simulink model "full_sim123deleteme"  (R2020b)
settings: Solver=ode1be  StartTime=0.0  StopTime=inf  RelTol=1e-3
InitFcn:
  | % Clear persistent variables in callback
  | clear all;
  | 
  | track = gen_track;
  | map = double(rgb2gray(imread('map.png')));%'iSpaceMapV2.0_50dpi.png')))*100/255;
  | 
  | % Load config data automatically
  | load("config.mat");
StartFcn:
  | % The event listener triggers when the signal updates, so we can just monitor one of the signals.
  | blk1 = 'full_sim/GUI_update';
  | 
  | event = 'PostOutputs';
  | listener = @updateApp;
  | 
  | % Create the listener
  | h1 = add_exec_event_listener(blk1, event, listener);
model workspace (MAT data in the model file):
  ResetMode : string (value not decoded)
  initX = -0.39
  initY = 0.33
  initYaw = 3.14159265359
libraries: simulink_extras x10, simulink x8, dspnetwork x6, pid_lib x2, sldrtlib x1
(part 2 of 2)

== matlab function full_sim123deleteme/EV3/Sensor Input Block/MATLAB Function ==
  data: pos input; rcx output; rcy output; lcx output; lcy output
function [rcx,rcy,lcx,lcy] = fcn(pos)
x = pos(1) + 0.06*cos(pos(3));
y = pos(2) + 0.06*sin(pos(3));
xScale = 1979.37;
yScale = -1925.58;
% xScale = 349.2718;
% yScale = -339.591;
topYReal = 2.936;
leftXReal = -1.9;
topYPixel = 943;
leftXPixel = 972;
% topYPixel = 168;
% leftXPixel = 166;
%pixel coords
x = round(leftXPixel + (xScale * (x-leftXReal)));
y = round(topYPixel + (yScale * (y-topYReal)));
lcy = floor(y-34*cos(pos(3)));
lcx = floor(x-34*sin(pos(3)));
rcy = floor(y+34*cos(pos(3)));
rcx = floor(x+34*sin(pos(3)));
% lcy = floor(y-6*cos(pos(3)));
% lcx = floor(x-6*sin(pos(3)));
% rcy = floor(y+6*cos(pos(3)));
% rcx = floor(x+6*sin(pos(3)));

end

== matlab function full_sim123deleteme/EV3/Sensor Input Block/left circle check ==
  data: map input; rli output; x input; y input; r input
function rli = circle(map,x,y,r)
%x and y are the coordinates of the center of the circle
%r is the radius of the circle
region = map(y-r:y+r, x-r:x+r); %matlab indexes the opposite of images, select s square around the circle 
[MX,MY] = meshgrid(-r:r, -r:r);
mask = MX.^2 + MY.^2 <= r^2;
rli = sum(sum(region.*double(mask))) / sum(sum(mask));%sum(sum(mask));
rli = round(rli * .7 + 10);
end

== matlab function full_sim123deleteme/EV3/Sensor Input Block/right circle check ==
  data: map input; rli output; x input; y input; r input
function rli = circle(map,x,y,r)
%x and y are the coordinates of the center of the circle
%r is the radius of the circle
region = map(y-r:y+r, x-r:x+r); %matlab indexes the opposite of images, select s square around the circle 
[MX,MY] = meshgrid(-r:r, -r:r);
mask = MX.^2 + MY.^2 <= r^2;
rli = sum(sum(region.*double(mask))) / sum(sum(mask));%sum(sum(mask));
rli = round(rli*.7 + 10);
end

== matlab function full_sim123deleteme/EV3/Sensor Input Block/Ultra_Sonic_Fcn ==
  data: pos input; other_pos input; ultrasonic output; omega input
function ultrasonic = Ultra_Sonic_Fcn(pos,other_pos,omega)
%NOTE: Assumed that position is being sent is in meters 

range_bound = 10;   %to solve for the upper and lower bounds
range_bound1 = 10;
range_bound2 = 10;
range_bound3 = 10;
range_bound4 = 10;

upp = 60;
mid = 30;
low = 20; 

value1 = 10;
value2 = 20;
value3 = 30; 

%find the distance between the two EVs
dist = other_pos(1:2) - pos(1:2);
   

%solve for hypotenuse between two vehicles. 
    dist_sq = (dist(1))^2 + (dist(2))^2; 
    hyp = sqrt(dist_sq); 
    
%hyp is in m need to convert to cm
    hyp = hyp*100; 
    
%since the positions are at the midpoint of the vehicles and not at the edges
    hyp = hyp -14; 

 %increase bounds with relation to how far away vehicle is 
  if hyp<=upp && hyp>=mid
      range_bound1 = range_bound+value1; 
  elseif hyp<=mid && hyp>=low
      range_bound1 = range_bound+value2; 
  elseif hyp<low
      range_bound1 = range_bound+value3; 
  end 
     

%find the trajected angle for the head motor
angle = atan2(dist(2), dist(1)); 

%need to find the angle of the head motor in relation to the rotation of the actual EV
head_ang = angle - pos(3); 
head_ang = -rad2deg(head_ang); 

%keeps angle within +/- 180 degrees
head_angle = mod(head_ang+180, 360) - 180; 

%find bounding region range using angle and radius --> 255 cm 
%check to see if the position of the other vehicle is within that bounding
%range. It if it is send that distance, if not send in 255 cm 

lower_bound = rad2deg(angdiff(deg2rad(range_bound1),deg2rad(head_angle)));  %must wrap bounds so that they stay within +/- 180 degrees
upper_bound = rad2deg(angdiff(deg2rad(-range_bound1),deg2rad(head_angle))); 
omeg = mod(omega+180, 360)-180; 

% 
%  %((pos(1)<=-0.40)&& (pos(2)<= 1.7)&&(pos(2)>=1.5)) %parking spot 3
%     %finding midpoints
%     % spot 3:
%     % -.8906, 1.72
%     % -.4953, 1.62
%     % -.8977, 1.5883
%     % -.5013, 1.4928
%     
%    up1 = [-0.8906 ; 1.72]; 
%    lo1 = [-0.8977 ; 1.5883];
%     
%     mid_z1 = (1.72+ 1.5883)/2; 
%     mid_x1 = ((-0.8977)+(-0.8906))/2;
%     
%     
%     %find true midpoint
%     midpoint1 = [mid_x1; mid_z1];
%     %find distance and hypotenuese
%     d1 = midpoint1 - pos(1:2); 
%     d_sq1 = (d1(1))^2 + (d1(2))^2; 
%     hype1 = sqrt(d_sq1); 
%     
%     %send in ultrasonic and convert from m to cm 
%     u1 = hype1*100; 
%     
%      %increase bounds with relation to how far away vehicle is 
%   if u1<=upp && u1>=mid
%       range_bound2 = range_bound+value1; 
%   elseif u1<=mid && u1>=low
%       range_bound2 = range_bound+value2; 
%   elseif u1<low
%       range_bound2 = range_bound+value3; 
%   end 
%     
%         %Parking Spot 3
%   %find the distance between the two EVs
%    %dist1 = midpoint1 - pos(1:2);
%    up_dist1 = up1 - pos(1:2);
%    lo_dist1 = lo1 - pos(1:2); 
% 
% %find the trajected angle for the head motor
%  %angle1 = atan2(dist1(2), dist1(1)); 
%  up_angle1 = atan2(up_dist1(2), up_dist1(1)); 
%  lo_angle1 = atan2(lo_dist1(2), lo_dist1(1)); 
% 
% %need to find the angle of the head motor in relation to the rotation of the actual EV
% %head_ang1 = angle1 - pos(3); 
% %head_ang1 = -rad2deg(head_ang1);
% 
% up_head1 = -rad2deg(up_angle1 - pos(3)); 
% lo_head1 = -rad2deg(lo_angle1 - pos(3)); 
% 
% %keeps angle within +/- 180 degrees
% %head_angle1 = mod(head_ang1+180, 360) - 180; 
% 
% up_head1 = mod(up_head1+180,360) - 180; 
% lo_head1 = mod(lo_head1+180, 360) - 180; 
% 
% lower_bound1 = rad2deg(angdiff(deg2rad(range_bound2),deg2rad(lo_head1)));  %must wrap bounds so that they stay within +/- 180 degrees
% upper_bound1 = rad2deg(angdiff(deg2rad(-range_bound2),deg2rad(up_head1))); 
% 
%  %((pos(1)<= -0.70)&&(pos(2)<=1.3)&&(pos(2)>=1.1)) %parking spot 2
%     %finding midpoints
%     % spot 2:
%     % -1.1672, 1.3082
%     % -.7708, 1.3162
%     % -1.1647, 1.0837
%     % -.7692, 1.0854
%     
%    up2 = [-1.1672 ; 1.3082]; 
%    lo2 = [-1.1647 ; 1.0837];
%           
%     mid_x2 = ((-1.1672)+(-1.1647))/2; 
%     mid_z2 = (1.3082+ 1.0837)/2; 
%    
%    
%     %find true midpoint
%     midpoint2 = [mid_x2 ; mid_z2];
%     %find distance and hypotenuese
%     d2 = midpoint2 - pos(1:2); 
%     d_sq2 = (d2(1))^2 + (d2(2))^2; 
%     hype2 = sqrt(d_sq2); 
%     
%     %send in ultrasonic and convert from m to cm 
%     u2= hype2*100; 
%     
%      %increase bounds with relation to how far away vehicle is 
%   if u2<=upp && u2>=mid
%       range_bound3 = range_bound+value1; 
%   elseif u2<=mid && u2>=low
%       range_bound3 = range_bound+value2; 
%   elseif u2<low
%       range_bound3 = range_bound+value3; 
%   end 
%     
%     %Parking Spot 2
% %find the distance between the two EVs
% %dist2 = midpoint2 - pos(1:2);
%    up_dist2 = up2 - pos(1:2);
%    lo_dist2 = lo2 - pos(1:2); 
% 
% %find the trajected angle for the head motor
% %angle2 = atan2(dist2(2), dist2(1)); 
%  up_angle2 = atan2(up_dist2(2), up_dist2(1)); 
%  lo_angle2 = atan2(lo_dist2(2), lo_dist2(1)); 
% 
% %need to find the angle of the head motor in relation to the rotation of the actual EV
% % head_ang2 = angle2 - pos(3); 
% % head_ang2 = -rad2deg(head_ang2); 
% up_head2 = -rad2deg(up_angle2 - pos(3)); 
% lo_head2 = -rad2deg(lo_angle2 - pos(3));
% 
% %keeps angle within +/- 180 degrees
% % head_angle2 = mod(head_ang2+180, 360) - 180; 
% up_head2 = mod(up_head2+180,360) - 180; 
% lo_head2 = mod(lo_head2+180, 360) - 180; 
% 
% lower_bound2 = rad2deg(angdiff(deg2rad(range_bound3),deg2rad(lo_head2)));  %must wrap bounds so that they stay within +/- 180 degrees
% upper_bound2 = rad2deg(angdiff(deg2rad(-range_bound3),deg2rad(up_head2))); 
% 
%   
%  %((pos(1)<=-0.80)&&(pos(2)<=0.90)&&(pos(2)>=0.70)) %parking spot 1
%     %finding midpoints
%     % spot 1: 
%     % -1.308, .9163
%     % -.9134, .9145
%     % -1.3115,.6954
%     % -.9171, .6931
%               
%    up3 = [-1.308 ; 0.9163]; 
%    lo3 = [-1.3115 ; 0.6954];
%    
%     mid_x3 = ((-1.308)+(-1.3115))/2; 
%     mid_z3 = (0.9163+ 0.6954)/2; 
%     
%     
%     %find true midpoint
%     midpoint3 = [mid_x3 ; mid_z3];
%     %find distance and hypotenuese
%     d3 = midpoint3 - pos(1:2); 
%     d_sq3 = (d3(1))^2 + (d3(2))^2; 
%     hype3 = sqrt(d_sq3); 
%     
%     %send in ultrasonic and convert from m to cm 
%     u3 = hype3*100;   
%     
%      %increase bounds with relation to how far away vehicle is 
%   if u3<=upp &&  u3>=mid
%       range_bound4 = range_bound+value1; 
%   elseif u3<=mid && u3>=low
%       range_bound4 = range_bound+value2; 
%   elseif u3<low
%       range_bound4 = range_bound+value3; 
%   end 
%     
%  %Parking Spot 1
% %find the distance between the two EVs
% %dist3 = midpoint3- pos(1:2);
% 
%    up_dist3 = up3 - pos(1:2);
%    lo_dist3 = lo3 - pos(1:2); 
%    
% %find the trajected angle for the head motor
% %angle3 = atan2(dist3(2), dist3(1)); 
%  up_angle3 = atan2(up_dist3(2), up_dist3(1)); 
%  lo_angle3 = atan2(lo_dist3(2), lo_dist3(1)); 
% 
% %need to find the angle of the head motor in relation to the rotation of the actual EV
% % head_ang3 = angle3 - pos(3);  
% % head_ang3 = -rad2deg(head_ang3); 
% 
% up_head3 = -rad2deg(up_angle3 - pos(3)); 
% lo_head3 = -rad2deg(lo_angle3 - pos(3));
% 
% %keeps angle within +/- 180 degrees
% % head_angle3 = mod(head_ang3+180, 360) - 180; 
% up_head3 = mod(up_head3+180,360) - 180; 
% lo_head3 = mod(lo_head3+180, 360) - 180; 
% 
% lower_bound3 = rad2deg(angdiff(deg2rad(range_bound4),deg2rad(lo_head3)));  %must wrap bounds so that they stay within +/- 180 degrees
% upper_bound3 = rad2deg(angdiff(deg2rad(-range_bound4),deg2rad(up_head3))); 
% 
% %when the angles wrap sometimes the bounds will need to change position
% %to match the bounding region 

ultrasonic = 255; 


if ((omeg>=lower_bound)&&(omeg<=upper_bound)&&(upper_bound>=lower_bound))||...
        (~((omeg>=upper_bound)&&(omeg<=lower_bound))&&(lower_bound>=upper_bound))
    
    %verify that the other_vehicle is the leader
%     if (pos(2)<=1 && other_pos(2)<=1 && other_pos(1)<= pos(1))||...    %bottom horizontal
%            (pos(2)>=1 &&  other_pos(2)>=1 && other_pos(1)>= pos(1) && dist(2)<=0.234)||...  %top horizontal
%            (other_pos(2)<=pos(2) && pos(1)<=1.870 && pos(1)>=1.5 && other_pos(1)<=1.870 && other_pos(1)>=1.5)||...  %-90 degree vertical
%            (other_pos(2)>=pos(2) && pos(1)<=-1.45 && pos(1)>=-1.65 && other_pos(1)<=-1.45 && other_pos(1)>=-1.65)   %90 degree vertical
            
    ultrasonic = min(ultrasonic, hyp); 
    
   % end 
end 

%     
% if ((omeg>=lower_bound1)&&(omeg<=upper_bound1)&&(upper_bound1>=lower_bound1))||...
%         (~((omeg>=upper_bound1)&&(omeg<=lower_bound1))&&(lower_bound1>=upper_bound1))
%     ultrasonic = min(ultrasonic, u1); 
% end 
%   
% 
% 
% if ((omeg>=lower_bound2)&&(omeg<=upper_bound2)&&(upper_bound2>=lower_bound2))||...
%         (~((omeg>=upper_bound2)&&(omeg<=lower_bound2))&&(lower_bound2>=upper_bound2))
%     ultrasonic = min(ultrasonic, u2); 
% end 
% 
% 
% if ((omeg>=lower_bound3)&&(omeg<=upper_bound3)&&(upper_bound3>=lower_bound3))||...
%         (~((omeg>=upper_bound3)&&(omeg<=lower_bound3))&&(lower_bound3>=upper_bound3))
%     ultrasonic = min(ultrasonic, u3);       
% end 

end
